simulink model "lab0"  (R2018a)
settings: Solver=FixedStepDiscrete  StartTime=0.0  StopTime=10.0  FixedStep=dt  RelTol=1e-3  EnableMultiTasking=on
values from neighbouring files (symbols this model uses):
  dt = 5e-3    (= 0.005)    [lab0.m]    (also in lab0_step.m)
libraries: legoev3lib x2
settings Model: SimulationMode=external  ExtModeTrigDuration=2  Creator=jacobdelrosario  LastModifiedBy=jacobdelrosario
settings SolverCC: PositivePriorityOrder=on
settings OptimizationCC: EnhancedBackFolding=on  PassReuseOutputArgsAs=Individual arguments  MaxStackSize=64  OptimizeBlockOrder=speed  DifferentSizesBufferReuse=on  OptimizationCustomize=off
settings DebuggingCC: ParameterTunabilityLossMsg=error
settings HardwareCC: ProdBitPerPointer=32  ProdBitPerSizeT=32  ProdBitPerPtrDiffT=32  ProdLargestAtomicInteger=Long  ProdWordSize=32  ProdHWDeviceType=ARM Compatible->ARM 9
settings SFSimCC: MATLABDynamicMemAlloc=off
settings RTWCC: SystemTargetFile=ert.tlc  HardwareBoard=LEGO MINDSTORMS EV3  TLCOptions="-aInlineSetEventsForThisBaseRateFcn=TLC_FALSE -aSuppressMultiTaskScheduler=TLC_FALSE  -aRateBasedStepFcn=0"  TemplateMakefile=ert_default_tmf  GenerateReport=on  Toolchain=Sourcery G++ Lite v2009q3  IncludeHyperlinkInReport=on  LaunchReport=on  GenerateTraceInfo=on  GenerateTraceReport=on  GenerateTraceReportSl=on  GenerateTraceReportSf=on  GenerateTraceReportEml=on
settings CodeAppCC: ForceParamTrailComments=on  IgnoreCustomStorageClasses=off  OperatorAnnotations=on  SimulinkDataObjDesc=on  SFDataObjDesc=on  InsertBlockDesc=on
settings ERTTargetCC: SupportContinuousTime=on  SupportVariableSizeSignals=on

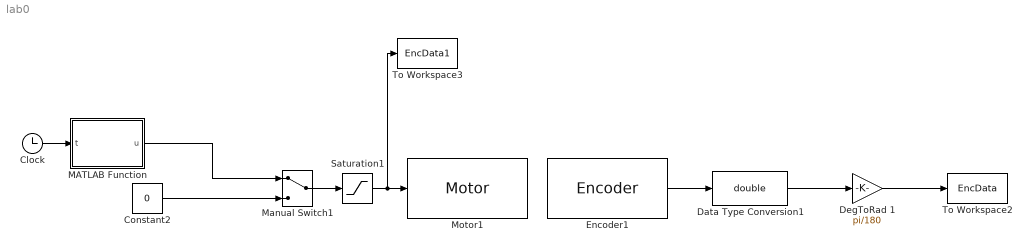
== system lab0 ==
  Clock : Clock
  Constant2 : Constant  Value=0  SampleTime=dt
  Data Type Conversion1 : DataTypeConversion  OutDataTypeStr=double
  DegToRad 1 : Gain  Gain=pi/180
  Encoder1 : legoev3lib/Encoder  portNumber=A  opMode=No reset  sampleTime=dt
      settings: SourceProductName=Simulink Support Package for LEGO MINDSTORMS EV3 Hardware  SourceProductBaseCode=LEGOEV3
  MATLAB Function : MATLAB Function  TreatAsAtomicUnit=on
  Manual Switch1 : ManualSwitch
  Motor1 : legoev3lib/Motor  sportNumber=A  sstopAction=Brake
  Saturation1 : Saturate  UpperLimit=100  LowerLimit=-100
  To Workspace2 : ToWorkspace  VariableName=EncData  SaveFormat=Structure With Time  SampleTime=dt
  To Workspace3 : ToWorkspace  VariableName=EncData1  SaveFormat=Structure With Time  SampleTime=dt
  wires:
  Manual Switch1/1 -> Saturation1/1
  Data Type Conversion1/1 -> DegToRad 1/1
  DegToRad 1/1 -> To Workspace2/1
  MATLAB Function/1(u) -> Manual Switch1/1
  Encoder1/1 -> Data Type Conversion1/1
  Constant2/1 -> Manual Switch1/2
  Saturation1/1 -> To Workspace3/1, Motor1/1
  Clock/1 -> MATLAB Function/1(t)

== matlab function lab0/MATLAB Function ==
  data: t input; u output

function u = fcn(t)

if (t>2)
    u = 100;
else
    u = 0;
end


end
